simulink model "uGrid_1PH_hd_ATD_prueba"  (R2018a)
settings: Solver=ode45  StartTime=0.0  StopTime=1.5  FixedStep=1e-4  MaxStep=1e-4  RelTol=1e-3
PreLoadFcn:
  | SimulinkInit
InitFcn:
  | SimulinkInit
values from neighbouring files (symbols this model uses):
  Ad = sysd.A    [SimulinkInit.m]
  b = 4.91    [parametros_BIO.m]
  Bd = sysd.B    [SimulinkInit.m]
  C = C1+C2+C3+Cl    (= 0.002654)    [SimulinkInit.m]    (also in parametros_BIO.m = 1)
  C1 = Cd(1,:)    [SimulinkInit.m]
  C2 = Cd(2,:)    [SimulinkInit.m]
  C3 = Cd(3,:)    [SimulinkInit.m]
  C4 = Cd(4,:)    [SimulinkInit.m]
  Cd = sysd.C    [SimulinkInit.m]
  K = 25    [parametros_BIO.m]    (also in uio_linear.m = K1+E*H)
  K1 = 1.15    [SimulinkInit.m]    (also in parametros_BIO.m = 9.66; uio_linear.m = K1')
  K11 = 0.8    [parametros_BIO.m]
  K2 = 1    [SimulinkInit.m]    (also in parametros_BIO.m = 6.97)
  K22 = 0.2    [parametros_BIO.m]
  K3 = 1    [SimulinkInit.m]    (also in parametros_BIO.m = 31.8)
  K33 = 0.23    [parametros_BIO.m]
  K4 = 15.1    [parametros_BIO.m]
  Kd = 0.02    [parametros_BIO.m]
  Kdc = 0.02    [parametros_BIO.m]
  Kf = 1    [parametros_BIO.m]
  Kh = 1.2    [parametros_BIO.m]
  Ks = 21.5    [parametros_BIO.m]
  Ksc = 3    [parametros_BIO.m]
  Kv = 1    [parametros_BIO.m]
  Sbin = 13.8    [parametros_BIO.m]
  Svin = 2.91    [parametros_BIO.m]
  T1 = 0.4    [parametros_BIO.m]
  T2 = 1    [parametros_BIO.m]
  T3 = 15    [parametros_BIO.m]
  T4 = 2.5    [parametros_BIO.m]
  T5 = 3.3    [parametros_BIO.m]
  Tao1 = 0.5    [SimulinkInit.m]
  Tcd = 0.2    [parametros_BIO.m]
  Tcr = 0.01    [parametros_BIO.m]
  Tf = 0.04    [parametros_BIO.m]
  tm = 1e-4    (= 0.0001)    [SimulinkInit.m]
  Tr = 950    [parametros_BIO.m]
  Tt = 450    [parametros_BIO.m]
  Ttd = 0.04    [parametros_BIO.m]
  Tv = 0.05    [parametros_BIO.m]
  V = 20    [parametros_BIO.m]
  wref = 70000    [parametros_BIO.m]
  X_acid = 1.2    [parametros_BIO.m]
  X_meth = 0.35    [parametros_BIO.m]
  Z = 3    [parametros_BIO.m]
undefined symbols (not defined in the file or in its folder): F1, F2, F3, F4, G, GF, H1, H2, H3, H4, Ion, K1U, K2U, K3U, K4U, Lithium, ss1, ss2
libraries: powerlib x58, dsparch4 x12, truetime x12, powerlib_meascontrol x4, simulink x1, electricdrivelib x1
(part 2 of 3)

== system uGrid_1PH_hd_ATD_prueba/CSI_Control_DIESEL ==
  V_measured : Inport
  I_measured : Inport  Port=2
  P_ref : Inport  Port=3
  Q_ref : Inport  Port=4
  Demux : Demux  Outputs=3
  Hw1 : dsparch4/Analog Filter Design  method=Bessel  filttype=Lowpass  N=4  Wlo=30*2*pi  Whi=80  Rp=2  Rs=80
  Hw3 : dsparch4/Analog Filter Design  method=Bessel  filttype=Lowpass  N=4  Wlo=30*2*pi  Whi=80  Rp=2  Rs=80
  Mux : Mux
  TTKernel_DIESEL : truetime/TrueTime Kernel  sfun=DIESEL_init  args=[]  ninputsoutputs=[4 3]  ntriggers=0  trigtype=falling  nwnodenbr=[]  clockoffsetdrift=[0 0]  schedoutput=on  battery=off  poweroutput=off
  D : Outport
  P_measure : Outport  Port=2
  Q_measure : Outport  Port=3
  wires:
  Mux/1 -> TTKernel_DIESEL/1
  Demux/3 -> Hw3/1
  Demux/2 -> Hw1/1
  TTKernel_DIESEL/1 -> Demux/1
  Demux/1 -> D/1
  Hw1/1 -> P_measure/1
  Hw3/1 -> Q_measure/1
  P_ref/1 -> Mux/3
  Q_ref/1 -> Mux/4
  I_measured/1 -> Mux/2
  V_measured/1 -> Mux/1

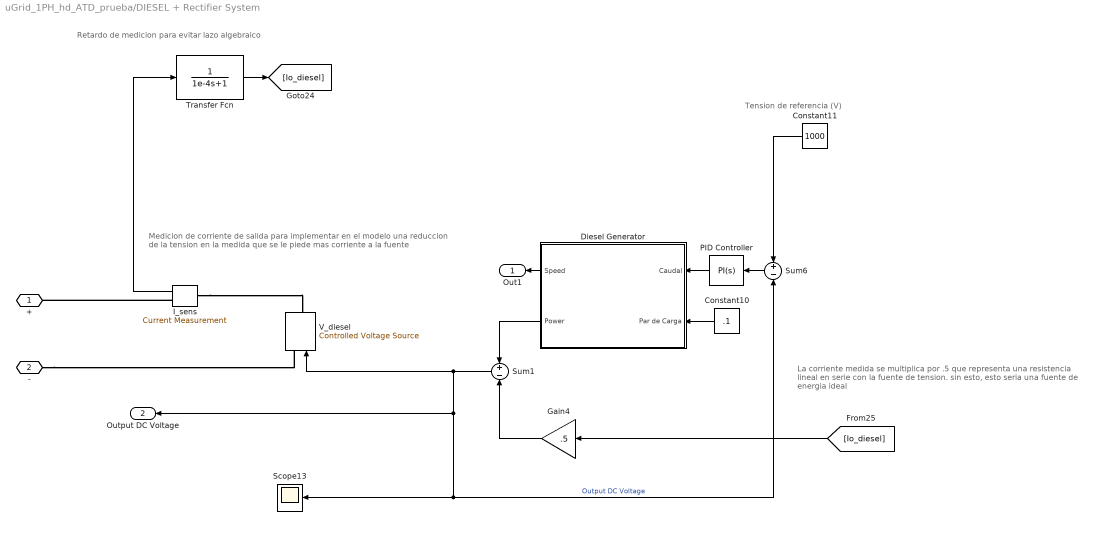
== system uGrid_1PH_hd_ATD_prueba/DIESEL + Rectifier System ==
  note: Tension de referencia (V)
  note: La corriente medida se multiplica por .5 que
      | representa una resistencia lineal en serie con
      | la fuente de tension. sin esto, esto seria una
      | fuente de energia ideal
  note: Medicion de corriente de salida para implementar
      | en el modelo una reduccion de la tension en la
      | medida que se le piede mas corriente a la fuente
  note: Retardo de medicion para evitar lazo algebraico
  Constant10 : Constant  Value=.1
  Constant11 : Constant  Value=1000
  Diesel Generator : Subsystem
  Gain4 : Gain  Gain=.5
  I_sens : powerlib/Measurements/Current Measurement  PhasorSimulation=off  OutputType=Complex  PSBequivalent=0
  PID Controller : simulink/Continuous/PID Controller  Controller=PI  TimeDomain=Continuous-time  SampleTime=-1  IntegratorMethod=Forward Euler  FilterMethod=Forward Euler  Form=Parallel  UseFilter=on  ControllerParametersSource=internal  P=0.00325909628031494  I=0.000326732379168699  D=0.00124823483730586  N=0.606508283225141  InitialConditionSource=internal  InitialConditionForIntegrator=0.248  InitialConditionForFilter=0.24  ExternalReset=none  LimitOutput=off  UpperSaturationLimit=inf  LowerSaturationLimit=-inf  LinearizeAsGain=on  AntiWindupMode=none  Kb=1  TrackingMode=off  Kt=1  PParamMin=[]  PParamMax=[]  IParamMin=[]  IParamMax=[]  DParamMin=[]  DParamMax=[]  NParamMin=[]  NParamMax=[]  KbParamMin=[]  KbParamMax=[]  KtParamMin=[]  KtParamMax=[]  POutMin=[]  POutMax=[]  IOutMin=[]  IOutMax=[]  DOutMin=[]  DOutMax=[]  NOutMin=[]  NOutMax=[]  KbOutMin=[]  KbOutMax=[]  KtOutMin=[]  KtOutMax=[]  IntegratorOutMin=[]  IntegratorOutMax=[]  FilterOutMin=[]  FilterOutMax=[]  SumOutMin=[]  SumOutMax=[]  SumI1OutMin=[]  SumI1OutMax=[]  SumI2OutMin=[]  SumI2OutMax=[]  SumI3OutMin=[]  SumI3OutMax=[]  SumDOutMin=[]  SumDOutMax=[]  SaturationOutMin=[]  SaturationOutMax=[]  IntegratorContinuousStateAttributes=''  IntegratorStateMustResolveToSignalObject=off  IntegratorRTWStateStorageClass=Auto  FilterContinuousStateAttributes=''  FilterStateMustResolveToSignalObject=off  FilterRTWStateStorageClass=Auto  DifferentiatorICPrevScaledInput=0  DifferentiatorOutMin=[]  DifferentiatorOutMax=[]  InitialConditionSetting=State (most efficient)  FilterDiffOutCoefMin=[]  FilterDiffOutCoefMax=[]  SumDenOutMin=[]  SumDenOutMax=[]  SumNumOutMin=[]  SumNumOutMax=[]  ReciprocalOutMin=[]  ReciprocalOutMax=[]  DivideOutMin=[]  DivideOutMax=[]  TunerSelectOption=Transfer Function Based (PID Tuner App)
  Scope13 : Scope
  Sum1 : Sum  Inputs=+-
  Sum6 : Sum  Inputs=+-
  Transfer Fcn : TransferFcn  Denominator=[1e-4 1]
  V_diesel : powerlib/Electrical Sources/Controlled Voltage Source  Initialize=on  Source_Type=AC  Amplitude=0  Phase=0  Frequency=0  Measurements=None
  + : PMIOPort  Side=Left
  - : PMIOPort  Port=2  Side=Left
  Out1 : Outport
  Output DC Voltage : Outport  Port=2
  wires:
  Sum1/1 -> Output DC Voltage/1, Sum6/2, Scope13/1, V_diesel/1  "Output DC Voltage"
  Transfer Fcn/1 -> [Io_diesel]
  I_sens/1 -> Transfer Fcn/1
  Diesel Generator/2(Power) -> Sum1/1
  Sum6/1 -> PID Controller/1
  Diesel Generator/1(Speed) -> Out1/1
  Gain4/1 -> Sum1/2
  Constant10/1 -> Diesel Generator/2(Par de Carga)
  Constant11/1 -> Sum6/1
  [Io_diesel] -> Gain4/1
  PID Controller/1 -> Diesel Generator/1(Caudal)
  connections:
  -/RConn1 -- V_diesel/LConn1
  I_sens/LConn1 -- V_diesel/RConn1
  I_sens/RConn1 -- +/RConn1

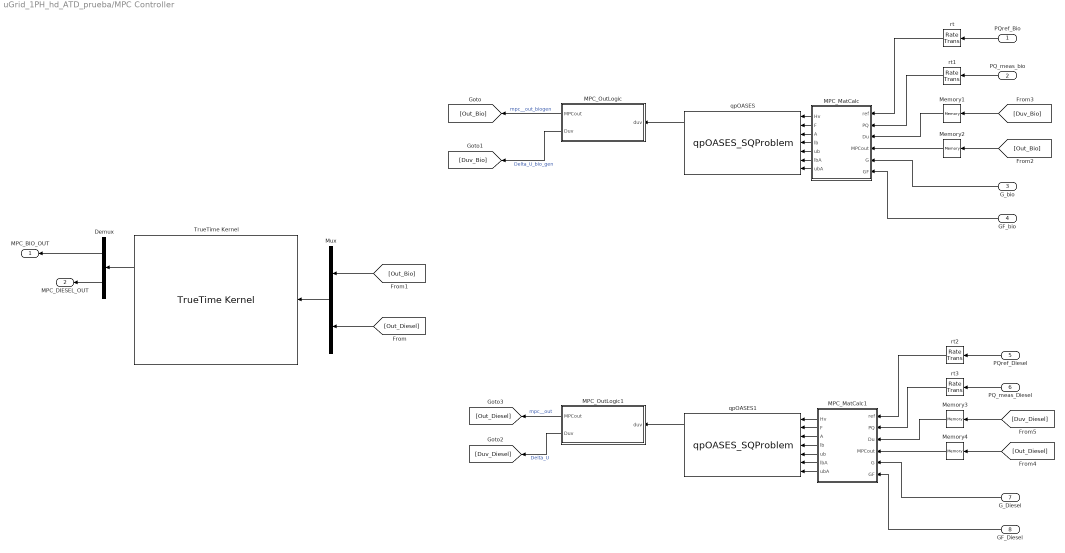
== system uGrid_1PH_hd_ATD_prueba/MPC Controller ==
  PQref_Bio : Inport
  PQ_meas_bio : Inport  Port=2
  G_bio : Inport  Port=3
  GF_bio : Inport  Port=4
  PQref_Diesel : Inport  Port=5
  PQ_meas_Diesel : Inport  Port=6
  G_Diesel : Inport  Port=7
  GF_Diesel : Inport  Port=8
  Demux : Demux  Outputs=2
  MPC_MatCalc : MATLAB Function  TreatAsAtomicUnit=on  SystemSampleTime=1e-3
      settings: MinAlgLoopOccurrences=on
  MPC_MatCalc1 : MATLAB Function  TreatAsAtomicUnit=on  SystemSampleTime=1e-3
      settings: MinAlgLoopOccurrences=on
  MPC_OutLogic : MATLAB Function  TreatAsAtomicUnit=on
      settings: MinAlgLoopOccurrences=on
  MPC_OutLogic1 : MATLAB Function  TreatAsAtomicUnit=on
      settings: MinAlgLoopOccurrences=on
  Memory{1..4} (4 alike) : Memory
  Mux : Mux  Inputs=2
  TrueTime Kernel : truetime/TrueTime Kernel  sfun=MPC_PQ_init  args=[]  ninputsoutputs=[4 4]  ntriggers=0  trigtype=falling  nwnodenbr=[]  clockoffsetdrift=[0 0]  schedoutput=on  battery=off  poweroutput=off
  qpOASES : S-Function  FunctionName=qpOASES_SQProblem  SFunctionDeploymentMode=off  EnableBusSupport=off
  qpOASES1 : S-Function  FunctionName=qpOASES_SQProblem  SFunctionDeploymentMode=off  EnableBusSupport=off
  rt{,1..3} (4 alike) : RateTransition  InitialCondition=[0 0]  OutPortSampleTime=1e-3
  MPC_BIO_OUT : Outport
  MPC_DIESEL_OUT : Outport  Port=2
  wires:
  MPC_MatCalc/7(ubA) -> qpOASES/7
  G_bio/1 -> MPC_MatCalc/5(G)
  MPC_MatCalc/4(lb) -> qpOASES/4
  MPC_MatCalc/6(lbA) -> qpOASES/6
  Memory1/1 -> MPC_MatCalc/3(Du)
  rt1/1 -> MPC_MatCalc/2(PQ)
  GF_bio/1 -> MPC_MatCalc/6(GF)
  PQ_meas_bio/1 -> rt1/1
  MPC_MatCalc/2(F) -> qpOASES/2
  Memory2/1 -> MPC_MatCalc/4(MPCout)
  MPC_MatCalc/5(ub) -> qpOASES/5
  MPC_MatCalc/3(A) -> qpOASES/3
  rt/1 -> MPC_MatCalc/1(ref)
  MPC_MatCalc/1(Hv) -> qpOASES/1
  PQref_Bio/1 -> rt/1
  MPC_MatCalc1/7(ubA) -> qpOASES1/7
  G_Diesel/1 -> MPC_MatCalc1/5(G)
  MPC_MatCalc1/4(lb) -> qpOASES1/4
  MPC_MatCalc1/6(lbA) -> qpOASES1/6
  Memory3/1 -> MPC_MatCalc1/3(Du)
  rt3/1 -> MPC_MatCalc1/2(PQ)
  GF_Diesel/1 -> MPC_MatCalc1/6(GF)
  PQ_meas_Diesel/1 -> rt3/1
  MPC_MatCalc1/2(F) -> qpOASES1/2
  Memory4/1 -> MPC_MatCalc1/4(MPCout)
  MPC_MatCalc1/5(ub) -> qpOASES1/5
  MPC_MatCalc1/3(A) -> qpOASES1/3
  rt2/1 -> MPC_MatCalc1/1(ref)
  MPC_MatCalc1/1(Hv) -> qpOASES1/1
  PQref_Diesel/1 -> rt2/1
  [Duv_Bio] -> Memory1/1
  [Out_Bio] -> Memory2/1
  [Duv_Diesel] -> Memory3/1
  [Out_Diesel] -> Memory4/1
  qpOASES1/1 -> MPC_OutLogic1/1(duv)
  qpOASES/1 -> MPC_OutLogic/1(duv)
  MPC_OutLogic1/2(Duv) -> [Duv_Diesel]  "Delta_U"
  MPC_OutLogic/1(MPCout) -> [Out_Bio]  "mpc__out_biogen"
  MPC_OutLogic1/1(MPCout) -> [Out_Diesel]  "mpc__out"
  Mux/1 -> TrueTime Kernel/1
  MPC_OutLogic/2(Duv) -> [Duv_Bio]  "Delta_U_bio_gen"
  TrueTime Kernel/1 -> Demux/1
  Demux/2 -> MPC_DIESEL_OUT/1
  Demux/1 -> MPC_BIO_OUT/1
  [Out_Diesel] -> Mux/2
  [Out_Bio] -> Mux/1

== system uGrid_1PH_hd_ATD_prueba/MeasureNode_I1 ==
  in : Inport
  Clock : Clock
  MATLAB Function : MATLAB Function  TreatAsAtomicUnit=on
  Pulse Generator1 : DiscretePulseGenerator  PulseType=Time based  Period=1e-4  PulseWidth=50  PhaseDelay=2e-4
  TrueTime Receive : truetime/TrueTime Receive  nwnbr=1  receiver=4  outdim=1  triggeroutput=on  senderoutput=off  lengthoutput=off  priorityoutput=off  timestampoutput=off  signalpoweroutput=off  msgIDoutput=off
  TrueTime Send : truetime/TrueTime Send  trigger=falling  nwnbr=1  sender=3  indim=1  recsource=internal  receiver=4  lengthsource=internal  length=10000  priosource=internal  prio=1  msgIDsource=internal  msgID=0  dynamicSegment=dynamic
  Out : Outport
  wires:
  Pulse Generator1/1 -> TrueTime Send/2
  TrueTime Receive/1 -> Out/1
  Clock/1 -> MATLAB Function/1(u1)
  MATLAB Function/1(y) -> TrueTime Send/1
  in/1 -> MATLAB Function/2(u2)

== system uGrid_1PH_hd_ATD_prueba/MeasureNode_I2 ==
  in : Inport
  Clock : Clock
  Delay : Delay  DelayLength=10
  MATLAB Function : MATLAB Function  TreatAsAtomicUnit=on
  Pulse Generator1 : DiscretePulseGenerator  PulseType=Time based  Period=1e-4  PulseWidth=50  PhaseDelay=1e-4
  TrueTime Receive : truetime/TrueTime Receive  nwnbr=1  receiver=2  outdim=1  triggeroutput=on  senderoutput=off  lengthoutput=off  priorityoutput=off  timestampoutput=off  signalpoweroutput=off  msgIDoutput=off
  TrueTime Send : truetime/TrueTime Send  trigger=falling  nwnbr=1  sender=1  indim=1  recsource=internal  receiver=2  lengthsource=internal  length=10000  priosource=internal  prio=1  msgIDsource=internal  msgID=0  dynamicSegment=dynamic
  Out : Outport
  wires:
  TrueTime Receive/1 -> Out/1
  Pulse Generator1/1 -> TrueTime Send/2
  Clock/1 -> MATLAB Function/1(u1)
  MATLAB Function/1(y) -> TrueTime Send/1
  in/1 -> Delay/1, MATLAB Function/2(u2)
  Delay/1 -> MATLAB Function/3(u3)

== system uGrid_1PH_hd_ATD_prueba/MeasureNode_I3 ==
  in : Inport
  Clock : Clock
  MATLAB Function : MATLAB Function  TreatAsAtomicUnit=on
  Pulse Generator1 : DiscretePulseGenerator  PulseType=Time based  Period=1e-4  PulseWidth=50  PhaseDelay=3e-4
  TrueTime Receive : truetime/TrueTime Receive  nwnbr=1  receiver=6  outdim=1  triggeroutput=on  senderoutput=off  lengthoutput=off  priorityoutput=off  timestampoutput=off  signalpoweroutput=off  msgIDoutput=off
  TrueTime Send : truetime/TrueTime Send  trigger=falling  nwnbr=1  sender=5  indim=1  recsource=internal  receiver=6  lengthsource=internal  length=10000  priosource=internal  prio=1  msgIDsource=internal  msgID=0  dynamicSegment=dynamic
  Out : Outport
  wires:
  in/1 -> MATLAB Function/2(u2)
  Pulse Generator1/1 -> TrueTime Send/2
  TrueTime Receive/1 -> Out/1
  Clock/1 -> MATLAB Function/1(u1)
  MATLAB Function/1(y) -> TrueTime Send/1

== system uGrid_1PH_hd_ATD_prueba/MeasureNode_I4 ==
  in : Inport
  Clock : Clock
  MATLAB Function : MATLAB Function  TreatAsAtomicUnit=on
  Pulse Generator1 : DiscretePulseGenerator  PulseType=Time based  Period=1e-4  PulseWidth=50  PhaseDelay=4e-4
  TrueTime Receive : truetime/TrueTime Receive  nwnbr=1  receiver=8  outdim=1  triggeroutput=on  senderoutput=off  lengthoutput=off  priorityoutput=off  timestampoutput=off  signalpoweroutput=off  msgIDoutput=off
  TrueTime Send : truetime/TrueTime Send  trigger=falling  nwnbr=1  sender=7  indim=1  recsource=internal  receiver=8  lengthsource=internal  length=10000  priosource=internal  prio=1  msgIDsource=internal  msgID=0  dynamicSegment=dynamic
  Out : Outport
  wires:
  Pulse Generator1/1 -> TrueTime Send/2
  TrueTime Receive/1 -> Out/1
  in/1 -> MATLAB Function/2(u2)
  MATLAB Function/1(y) -> TrueTime Send/1
  Clock/1 -> MATLAB Function/1(u1)

== system uGrid_1PH_hd_ATD_prueba/Subsystem ==
  Battery : electricdrivelib/Extra Sources/Battery  BatType=Lithium-Ion  ShowTempParam=off  ThermalPreset=no  ShowAgeParam=off  NomV=1000  NomQ=20  SOC=100  Batt_Tr=10e-3  PresetModel=off  MaxQ=1  MinV=825  FullV=1280.3859  Dis_rate=200  R=50e-3  Normal_OP=0.90435  expZone="[1188.4244    0.049130435]"  current=[6.5 13 32.5 50]  Units=Time  Tci=20  NomT=20  T2=-30  MaxQ2=4.8  FullV2=7.1  Normal_OP2=5.655  expZone2="[6.58           1]"  Rca=0.6  ti=2000  Dp=0  Neq0=0  Tsim=1e6  Ta1=25  Qeol=5.4*0.9  Reol=0.013333*1.2  Char_age=[2.3478, 3]  Dis_age=[2.3478, 10]  N1=1500  N2=10500  N3=1000  N4=1400  Ta2=45  N5=950
  Constant2 : Constant  Value=1000
  Constant4 : Constant  Value=25
  Controlled Current Source : powerlib/Electrical Sources/Controlled Current Source  Initialize=on  Source_Type=AC  Amplitude=0  Phase=0  Frequency=0  Measurements=None
  Gain3 : Gain  Gain=1/10
  PV panel1 : Subsystem
      mask Display: image('panel.jpg')
  Rcable : powerlib/Elements/Series RLC Branch  LConnTagsString=__new0  RConnTagsString=__new0  BranchType=R  Resistance=1e-3  Inductance=1e-3  SetiL0=off  InitialCurrent=0  Capacitance=1e-6  Setx0=off  InitialVoltage=0  Measurements=None
  Rin2 : powerlib/Elements/Series RLC Branch  LConnTagsString=__new0  RConnTagsString=__new0  BranchType=C  Resistance=.001  Inductance=0  SetiL0=off  InitialCurrent=0  Capacitance=1000e-6  Setx0=off  InitialVoltage=0  Measurements=None
  + : PMIOPort  Side=Left
  - : PMIOPort  Port=2  Side=Left
  Out1 : Outport
  wires:
  PV panel1/1(I) -> Gain3/1
  Gain3/1 -> Controlled Current Source/1
  Battery/1 -> Out1/1
  Constant4/1 -> PV panel1/3(Top)
  Constant2/1 -> PV panel1/2(G)
  [V] -> PV panel1/1(V)
  connections:
  Rcable/RConn1 -- +/RConn1
  Battery/LConn1 -- Controlled Current Source/RConn1 -- Rcable/LConn1 -- Rin2/LConn1
  Battery/LConn2 -- -/RConn1 -- Rin2/RConn1 -- Controlled Current Source/LConn1

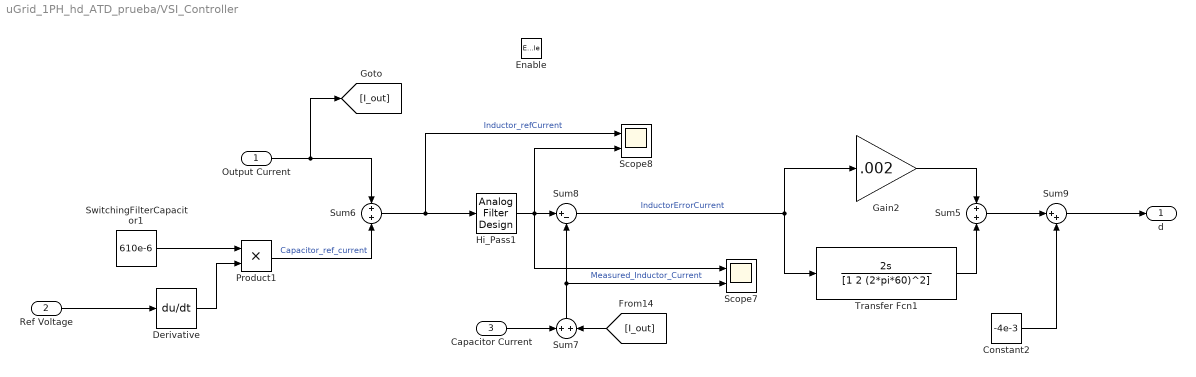
== system uGrid_1PH_hd_ATD_prueba/VSI_Controller ==
  Output Current : Inport
  Ref Voltage : Inport  Port=2
  Capacitor Current : Inport  Port=3
  Enable : EnablePort
  Constant2 : Constant  Value=-4e-3
  Derivative : Derivative  CoefficientInTFapproximation=1e-3
  Gain2 : Gain  Gain=.002
  Hi_Pass1 : dsparch4/Analog Filter Design  method=Bessel  filttype=Highpass  N=1  Wlo=1*2*pi  Whi=80  Rp=2  Rs=40
  Product1 : Product
  Scope7 : Scope  NumInputPorts=2
  Scope8 : Scope  NumInputPorts=2
  Sum5 : Sum  Inputs=+|+
  Sum6 : Sum  Inputs=+|+
  Sum7 : Sum  Inputs=+|+
  Sum8 : Sum  Inputs=|+-
  Sum9 : Sum  Inputs=|++
  SwitchingFilterCapacitor1 : Constant  Value=610e-6
  Transfer Fcn1 : TransferFcn  Numerator=[2 0]  Denominator=[1 2 (2*pi*60)^2]
  d : Outport
  wires:
  Derivative/1 -> Product1/2
  Sum6/1 -> Hi_Pass1/1, Scope8/1  "Inductor_refCurrent"
  Sum8/1 -> Transfer Fcn1/1, Gain2/1  "InductorErrorCurrent"
  Ref Voltage/1 -> Derivative/1
  Constant2/1 -> Sum9/2
  Capacitor Current/1 -> Sum7/1
  Transfer Fcn1/1 -> Sum5/2
  Output Current/1 -> Sum6/1, [I_out]
  [I_out] -> Sum7/2
  Gain2/1 -> Sum5/1
  SwitchingFilterCapacitor1/1 -> Product1/1
  Hi_Pass1/1 -> Scope8/2, Sum8/1, Scope7/1
  Product1/1 -> Sum6/2  "Capacitor_ref_current"
  Sum9/1 -> d/1
  Sum5/1 -> Sum9/1
  Sum7/1 -> Scope7/2, Sum8/2  "Measured_Inductor_Current"

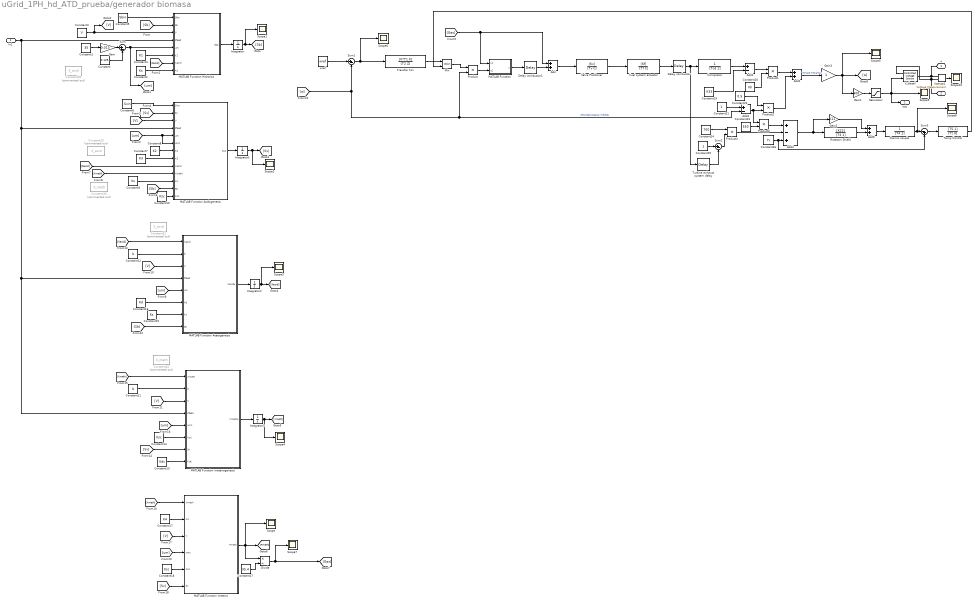
== system uGrid_1PH_hd_ATD_prueba/generador biomasa ==
  In1 : Inport
  Add : Sum
  Add1 : Sum  Inputs=+-
  Add2 : Sum
  Add3 : Sum  Inputs=+-
  Add4 : Sum  Inputs=+-+
  Add5 : Sum
  Compresor : TransferFcn  Denominator=[Tcd 1]
  Constant : Constant  Value=0.129
  Constant1 : Constant  Value=35
  Constant10 : Constant  Value=Ksc
  Constant11 : Constant  Value=b
  Constant12 : Constant  Value=b
  Constant13 : Constant  Value=Kdc
  Constant14 : Constant  Value=Ksc
  Constant15 : Constant  Value=Ks
  Constant16 : Constant  Value=Kd
  Constant17 : Constant  Value=K4
  Constant18 : Constant  Value=Ksc
  Constant19 : Constant  Value=K33
  Constant2 : Constant  Value=Ks
  Constant20 : Constant  Value=Kh
  Constant21 : Constant
  Constant22 : Constant  Value=0.5
  Constant23 : Constant  Value=550
  Constant24 : Constant  Value=700
  Constant25 : Constant
  Constant26 : Constant  Value=Tr
  Constant27 : Constant  Value=35.4
  Constant28 : Constant  Commented=on  Value=X_acid
  Constant29 : Constant  Commented=on  Value=X_acid
  Constant3 : Constant  Value=V
  Constant30 : Constant  Commented=on  Value=X_meth
  Constant31 : Constant  Commented=on  Value=X_acid
  Constant32 : Constant  Commented=on  Value=X_meth
  Constant4 : Constant  Value=K1
  Constant5 : Constant  Value=Sbin
  Constant6 : Constant  Value=Svin
  Constant7 : Constant  Value=K3
  Constant8 : Constant  Value=K2
  Constant9 : Constant  Value=Ks
  Delay combustor : TransportDelay  DelayTime=Tcr
  Delay combustor1 : TransportDelay  DelayTime=0
  Divide : Product  Inputs=*/
  Fuel system actuator : TransferFcn  Numerator=[Kf]  Denominator=[Tf C]
  Gain : Gain  Gain=0.013
  Gain1 : Gain  Gain=900
  Gain2 : Gain  Gain=K11
  Gain3 : Gain
  Integrator : Integrator
  Integrator1 : Integrator
  Integrator2 : Integrator  InitialCondition=1.2
  Integrator3 : Integrator  InitialCondition=0.35
  MATLAB Function : MATLAB Function  TreatAsAtomicUnit=on
  MATLAB Function Acetogenesis : MATLAB Function  TreatAsAtomicUnit=on
  MATLAB Function Acidogenesis : MATLAB Function  TreatAsAtomicUnit=on
  MATLAB Function Hidrolisis : MATLAB Function  TreatAsAtomicUnit=on
  MATLAB Function metano : MATLAB Function  TreatAsAtomicUnit=on
  MATLAB Function metanogenesis : MATLAB Function  TreatAsAtomicUnit=on
  Min : MinMax  Inputs=2
  Product{,1..4} (5 alike) : Product
  Rotation Shield : TransferFcn  Numerator=[K22]  Denominator=[T3 1]
  Saturation : Saturate  UpperLimit=1000  LowerLimit=0
  Scope{,1..10} (11 alike) : Scope
  Sum : Sum  Inputs=|+-
  Sum1 : Sum  Inputs=|+-
  Sum2 : Sum  Inputs=|+-
  Sum3 : Sum  Inputs=|-+
  Temp Control : TransferFcn  Numerator=[T5 1]  Denominator=[Tt 0]
  Transfer Fcn : TransferFcn  Numerator=[K*T1 K]  Denominator=[T2 Z]
  Turbine exhaust system delay : TransportDelay  DelayTime=Ttd
  V_diesel : powerlib/Electrical Sources/Controlled Voltage Source  Initialize=on  Source_Type=DC  Amplitude=0  Phase=0  Frequency=0  Measurements=None
  Valve Positioner : TransferFcn  Numerator=[Kv]  Denominator=[Tv C]
  Vsensa1 : powerlib/Measurements/Voltage Measurement  PhasorSimulation=off  OutputType=Complex  PSBequivalent=0
  thermo couple : TransferFcn  Denominator=[T4 1]
  wref : Constant  Value=wref
  + : PMIOPort  Side=Left
  - : PMIOPort  Port=2  Side=Left
  Vdc : Outport
  wires:
  MATLAB Function metano/1(Fmeth) -> Divide/1, Scope/1, [Fmeth]
  Sum/1 -> [um], MATLAB Function Hidrolisis/5(um)
  Constant16/1 -> MATLAB Function Acetogenesis/6(Kd)
  Temp Control/1 -> Min/2
  Integrator/1 -> Scope1/1, [Sb]
  Gain3/1 -> Gain1/1, Scope5/1, [w]
  Sum1/1 -> Transfer Fcn/1, Scope6/1
  [Sb] -> MATLAB Function Acetogenesis/8(Sb)
  [Sv] -> MATLAB Function metanogenesis/7(Sv)
  Add4/1 -> Rotation Shield/1, Gain2/1
  Constant8/1 -> MATLAB Function Acidogenesis/7(K2)
  Constant24/1 -> Product4/1
  [V] -> MATLAB Function Acetogenesis/3(V)
  Constant23/1 -> Product3/2
  Constant27/1 -> Divide/2
  [Sb] -> MATLAB Function Acidogenesis/12(Sb)
  Integrator3/1 -> Scope4/1, [Xmeth]
  Integrator2/1 -> Scope3/1, [Xacid]
  Divide/1 -> Scope7/1, [Gas]
  Constant7/1 -> MATLAB Function Acidogenesis/8(K3)
  Delay combustor/1 -> Turbine exhaust system delay/1, Compresor/1
  [V] -> MATLAB Function Acidogenesis/3(V)
  Constant12/1 -> MATLAB Function Acetogenesis/2(b)
  Sum2/1 -> Product4/2
  [V] -> MATLAB Function metanogenesis/3(V)
  Gain/1 -> Sum/1
  Product/1 -> MATLAB Function/2(u2)
  [w] -> Product/2, Add3/2, Sum1/2  "velocidad angular medida"
  Constant6/1 -> MATLAB Function Acidogenesis/1(Svin)
  wref/1 -> Sum1/1
  [Gas] -> MATLAB Function/1(u1), Add/1
  [Sv] -> MATLAB Function metano/6(Sv)
  MATLAB Function Hidrolisis/1(Sbp) -> Integrator/1
  Turbine exhaust system delay/1 -> Sum2/2
  MATLAB Function Acetogenesis/1(Xacidp) -> Integrator2/1
  Constant/1 -> Sum/2
  Constant18/1 -> MATLAB Function metano/5(Ksc)
  In1/1 -> MATLAB Function Acidogenesis/4(Ffeed), MATLAB Function metanogenesis/4(Ffeed), MATLAB Function Acetogenesis/4(Ffeed), MATLAB Function Hidrolisis/4(Ffeed)
  Add3/1 -> Product3/1, Product2/2
  [um] -> MATLAB Function Acetogenesis/5(um)
  Product3/1 -> Add4/1
  Constant15/1 -> MATLAB Function Acetogenesis/7(Ks)
  thermo couple/1 -> Scope8/1, Sum3/1
  Fuel system actuator/1 -> Delay combustor/1
  Add/1 -> Valve Positioner/1
  Add5/1 -> thermo couple/1
  Gain2/1 -> Add5/1
  Constant22/1 -> Product2/1
  [um] -> MATLAB Function metano/4(umc)
  Compresor/1 -> Add1/1
  Constant10/1 -> MATLAB Function Acidogenesis/13(Ksc)
  [um] -> MATLAB Function Acidogenesis/6(umc), MATLAB Function Acidogenesis/5(um)
  Constant9/1 -> MATLAB Function Acidogenesis/11(Ks)
  Constant1/1 -> Gain/1
  Constant13/1 -> MATLAB Function metanogenesis/8(Kdc)
  Constant26/1 -> Sum3/2, Add4/3
  Integrator1/1 -> Scope2/1, [Sv]
  [Xmeth] -> MATLAB Function metanogenesis/1(Xmeth)
  Add2/1 -> Gain3/1  "Torque mecánico"
  MATLAB Function/1(y) -> Delay combustor1/1
  Saturation/1 -> Vdc/1, V_diesel/1, Scope9/1
  [Sb] -> MATLAB Function Hidrolisis/2(Sb)
  Min/1 -> Product/1
  Constant3/1 -> [V], MATLAB Function Hidrolisis/3(V)
  MATLAB Function Acidogenesis/1(Svp) -> Integrator1/1
  Constant5/1 -> MATLAB Function Hidrolisis/1(Sbin)
  Constant20/1 -> Product1/2
  [Xmeth] -> MATLAB Function Acidogenesis/10(Xmeth)
  Sum3/1 -> Temp Control/1
  Gain1/1 -> Saturation/1
  Constant21/1 -> Add3/1
  Constant25/1 -> Sum2/1
  Product2/1 -> Add2/2
  [Xacid] -> MATLAB Function Acidogenesis/9(Xacid)
  Valve Positioner/1 -> Fuel system actuator/1
  Constant4/1 -> MATLAB Function Hidrolisis/6(K1)
  Constant11/1 -> MATLAB Function metanogenesis/2(b)
  Rotation Shield/1 -> Add5/2
  Add1/1 -> Product1/1
  [Sv] -> MATLAB Function Acidogenesis/2(Sv)
  [Xacid] -> MATLAB Function Acetogenesis/1(Xacid)
  Constant19/1 -> Add1/2
  Product1/1 -> Add2/1
  Transfer Fcn/1 -> Min/1
  Delay combustor1/1 -> Add/2
  [um] -> MATLAB Function metanogenesis/5(umc)
  MATLAB Function metanogenesis/1(Xmethp) -> Integrator3/1
  Constant14/1 -> MATLAB Function metanogenesis/6(Ksc)
  Product4/1 -> Add4/2
  Constant2/1 -> MATLAB Function Hidrolisis/8(Ks)
  Constant17/1 -> MATLAB Function metano/2(K4)
  [V] -> MATLAB Function metano/3(V)
  [Xmeth] -> MATLAB Function metano/1(Xmeth)
  [Xacid] -> MATLAB Function Hidrolisis/7(Xacid)
  Vsensa1/1 -> Scope10/1
  connections:
  V_diesel/RConn1 -- Vsensa1/LConn1 -- +/RConn1
  V_diesel/LConn1 -- Vsensa1/LConn2 -- -/RConn1

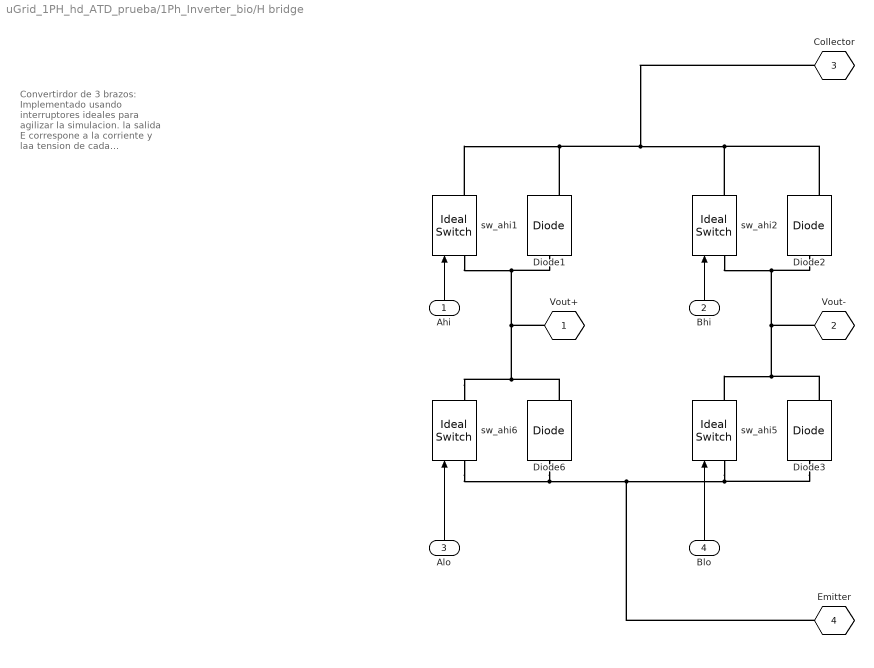
== system uGrid_1PH_hd_ATD_prueba/1Ph_Inverter_bio/H bridge ==
  note: Convertirdor de 3 brazos:
      |
      | Implementado usando interruptores
      | ideales para agilizar la simulacion.
      | la salida E correspone a la corriente y laa
      | tension de cada componente
      | (sea interruptor o diodo) y su respectiva
      | corriente. no tienen puerto de salida ya que no
      | son relevantes para lo que se desea simular.
      |
      | si g=0 interruptor no conduce.
      | si g=1 interruptor conduce.
      |
      | conmutacion ocurre instantaneamente sin
      | retardo.
  Ahi : Inport
  Bhi : Inport  Port=2
  Alo : Inport  Port=3
  Blo : Inport  Port=4
   sw_ahi{1..2,5..6} (4 alike) : powerlib/Power Electronics/Ideal Switch  Ron=0.1  Lon=0  IC=0  Rs=1e6  Cs=10e-12  Measurements=on
  Diode{1..3,6} (4 alike) : powerlib/Power Electronics/Diode  Ron=.2  Lon=0  Vf=0.8  IC=0  UseSnubber=0  Rs=0  Cs=0  Measurements=on
  " Vout+" : PMIOPort  Tag=PMCPort  Side=Right
  Vout- : PMIOPort  Tag=PMCPort  Port=2  Side=Right
  Collector : PMIOPort  Tag=PMCPort  Port=3  Side=Right
  Emitter : PMIOPort  Tag=PMCPort  Port=4  Side=Right
  wires:
  Alo/1 -> " sw_ahi6"/1
  Ahi/1 -> " sw_ahi1"/1
  Blo/1 -> " sw_ahi5"/1
  Bhi/1 -> " sw_ahi2"/1
  connections:
  Diode3/RConn1 -- Vout-/RConn1 -- " sw_ahi2"/LConn1 -- Diode2/LConn1 -- " sw_ahi5"/RConn1
  Diode3/LConn1 -- Emitter/RConn1 -- Diode6/LConn1 -- " sw_ahi6"/LConn1 -- " sw_ahi5"/LConn1
  Diode2/RConn1 -- Collector/RConn1 -- " sw_ahi1"/RConn1 -- Diode1/RConn1 -- " sw_ahi2"/RConn1
  " sw_ahi6"/RConn1 -- Diode6/RConn1 -- " Vout+"/RConn1 -- Diode1/LConn1 -- " sw_ahi1"/LConn1

== system uGrid_1PH_hd_ATD_prueba/1Ph_Inverter_bio/Io_measure ==
  A_current : Inport
  Enable : EnablePort
  Hw1 : dsparch4/Analog Filter Design  method=Bessel  filttype=Lowpass  N=2  Wlo=7000*2*pi  Whi=80  Rp=2  Rs=80
  Transfer Fcn : TransferFcn  Denominator=[1e-6 1]
  Out1 : Outport
  wires:
  Transfer Fcn/1 -> Hw1/1
  A_current/1 -> Transfer Fcn/1
  Hw1/1 -> Out1/1

== system uGrid_1PH_hd_ATD_prueba/1Ph_Inverter_bio/Subsystem ==
  Din : Inport
  Enable : EnablePort
  Gain : Gain  Gain=15
  PWM Generator (DC-DC) : powerlib_meascontrol/Pulse & Signal Generators/PWM Generator (DC-DC)  Fsw=f_sw  Ts=samp_f
  Steper1 : Subsystem
  Steper3 : Subsystem
  not_pwm : MATLAB Function  TreatAsAtomicUnit=on
  nPWM : Outport
  PWM : Outport  Port=2
  wires:
  not_pwm/1(y) -> Steper3/1(In1)
  Steper3/1(Out1) -> nPWM/1
  Gain/1 -> Steper1/1(In1), not_pwm/1(u)
  Din/1 -> PWM Generator (DC-DC)/1
  PWM Generator (DC-DC)/1 -> Gain/1
  Steper1/1(Out1) -> PWM/1

== system uGrid_1PH_hd_ATD_prueba/1Ph_Inverter_bio/Subsystem1 ==
  A_volts : Inport
  Enable : EnablePort
  Hw4 : dsparch4/Analog Filter Design  method=Bessel  filttype=Lowpass  N=2  Wlo=7000*2*pi  Whi=80  Rp=2  Rs=80
  Transfer Fcn1 : TransferFcn  Denominator=[1e-6 1]
  Out1 : Outport
  wires:
  A_volts/1 -> Transfer Fcn1/1
  Transfer Fcn1/1 -> Hw4/1
  Hw4/1 -> Out1/1

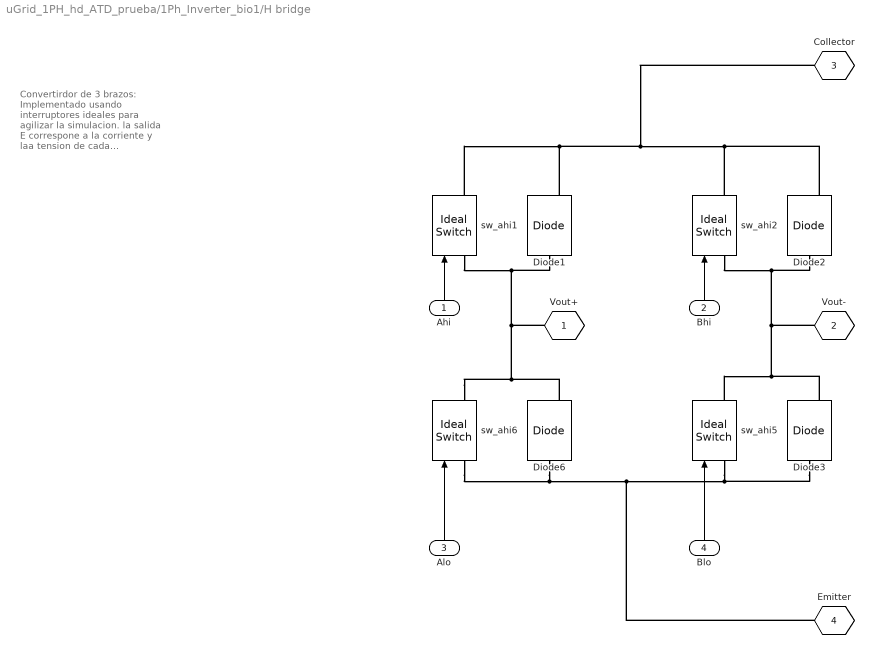
== system uGrid_1PH_hd_ATD_prueba/1Ph_Inverter_bio1/H bridge ==
  note: Convertirdor de 3 brazos:
      |
      | Implementado usando interruptores
      | ideales para agilizar la simulacion.
      | la salida E correspone a la corriente y laa
      | tension de cada componente
      | (sea interruptor o diodo) y su respectiva
      | corriente. no tienen puerto de salida ya que no
      | son relevantes para lo que se desea simular.
      |
      | si g=0 interruptor no conduce.
      | si g=1 interruptor conduce.
      |
      | conmutacion ocurre instantaneamente sin
      | retardo.
  Ahi : Inport
  Bhi : Inport  Port=2
  Alo : Inport  Port=3
  Blo : Inport  Port=4
   sw_ahi{1..2,5..6} (4 alike) : powerlib/Power Electronics/Ideal Switch  Ron=0.1  Lon=0  IC=0  Rs=1e6  Cs=10e-12  Measurements=on
  Diode{1..3,6} (4 alike) : powerlib/Power Electronics/Diode  Ron=.2  Lon=0  Vf=0.8  IC=0  UseSnubber=0  Rs=0  Cs=0  Measurements=on
  " Vout+" : PMIOPort  Tag=PMCPort  Side=Right
  Vout- : PMIOPort  Tag=PMCPort  Port=2  Side=Right
  Collector : PMIOPort  Tag=PMCPort  Port=3  Side=Right
  Emitter : PMIOPort  Tag=PMCPort  Port=4  Side=Right
  wires:
  Alo/1 -> " sw_ahi6"/1
  Ahi/1 -> " sw_ahi1"/1
  Blo/1 -> " sw_ahi5"/1
  Bhi/1 -> " sw_ahi2"/1
  connections:
  Diode3/RConn1 -- Vout-/RConn1 -- " sw_ahi2"/LConn1 -- Diode2/LConn1 -- " sw_ahi5"/RConn1
  Diode3/LConn1 -- Emitter/RConn1 -- Diode6/LConn1 -- " sw_ahi6"/LConn1 -- " sw_ahi5"/LConn1
  Diode2/RConn1 -- Collector/RConn1 -- " sw_ahi1"/RConn1 -- Diode1/RConn1 -- " sw_ahi2"/RConn1
  " sw_ahi6"/RConn1 -- Diode6/RConn1 -- " Vout+"/RConn1 -- Diode1/LConn1 -- " sw_ahi1"/LConn1

== system uGrid_1PH_hd_ATD_prueba/1Ph_Inverter_bio1/Ic Measure ==
  Ic : Inport
  Enable : EnablePort
  Hw5 : dsparch4/Analog Filter Design  method=Bessel  filttype=Lowpass  N=2  Wlo=7000*2*pi  Whi=80  Rp=2  Rs=80
  Transfer Fcn2 : TransferFcn  Denominator=[1e-6 1]
  Out1 : Outport
  wires:
  Transfer Fcn2/1 -> Hw5/1
  Ic/1 -> Transfer Fcn2/1
  Hw5/1 -> Out1/1

== system uGrid_1PH_hd_ATD_prueba/1Ph_Inverter_bio1/Io_measure ==
  A_current : Inport
  Enable : EnablePort
  Hw2 : dsparch4/Analog Filter Design  method=Bessel  filttype=Lowpass  N=2  Wlo=7000*2*pi  Whi=80  Rp=2  Rs=80
  Transfer Fcn : TransferFcn  Denominator=[1e-6 1]
  Out1 : Outport
  wires:
  Transfer Fcn/1 -> Hw2/1
  Hw2/1 -> Out1/1
  A_current/1 -> Transfer Fcn/1

== system uGrid_1PH_hd_ATD_prueba/1Ph_Inverter_bio1/Steper1 ==
  In1 : Inport
  Product : Product
  Step : Step  Time=st_time  SampleTime=samp_f
  Out1 : Outport
  wires:
  Step/1 -> Product/2
  In1/1 -> Product/1
  Product/1 -> Out1/1

== system uGrid_1PH_hd_ATD_prueba/1Ph_Inverter_bio1/Steper3 ==
  In1 : Inport
  Product : Product
  Step : Step  Time=st_time  SampleTime=samp_f
  Out1 : Outport
  wires:
  Product/1 -> Out1/1
  In1/1 -> Product/1
  Step/1 -> Product/2

== system uGrid_1PH_hd_ATD_prueba/1Ph_Inverter_bio1/Vo_measure ==
  A_volts : Inport
  Enable : EnablePort
  Hw6 : dsparch4/Analog Filter Design  method=Bessel  filttype=Lowpass  N=2  Wlo=7000*2*pi  Whi=80  Rp=2  Rs=80
  Transfer Fcn1 : TransferFcn  Denominator=[1e-6 1]
  Out1 : Outport
  wires:
  Transfer Fcn1/1 -> Hw6/1
  Hw6/1 -> Out1/1
  A_volts/1 -> Transfer Fcn1/1

== system uGrid_1PH_hd_ATD_prueba/1Ph_Inverter_diesel/H bridge ==
  note: Convertirdor de 3 brazos:
      |
      | Implementado usando interruptores
      | ideales para agilizar la simulacion.
      | la salida E correspone a la corriente y laa
      | tension de cada componente
      | (sea interruptor o diodo) y su respectiva
      | corriente. no tienen puerto de salida ya que no
      | son relevantes para lo que se desea simular.
      |
      | si g=0 interruptor no conduce.
      | si g=1 interruptor conduce.
      |
      | conmutacion ocurre instantaneamente sin
      | retardo.
  Ahi : Inport
  Bhi : Inport  Port=2
  Alo : Inport  Port=3
  Blo : Inport  Port=4
   sw_ahi{1..2,5..6} (4 alike) : powerlib/Power Electronics/Ideal Switch  Ron=0.1  Lon=0  IC=0  Rs=1e6  Cs=10e-12  Measurements=on
  Diode{1..3,6} (4 alike) : powerlib/Power Electronics/Diode  Ron=.2  Lon=0  Vf=0.8  IC=0  UseSnubber=0  Rs=0  Cs=0  Measurements=on
  " Vout+" : PMIOPort  Tag=PMCPort  Side=Right
  Vout- : PMIOPort  Tag=PMCPort  Port=2  Side=Right
  Collector : PMIOPort  Tag=PMCPort  Port=3  Side=Right
  Emitter : PMIOPort  Tag=PMCPort  Port=4  Side=Right
  wires:
  Bhi/1 -> " sw_ahi2"/1
  Blo/1 -> " sw_ahi5"/1
  Ahi/1 -> " sw_ahi1"/1
  Alo/1 -> " sw_ahi6"/1
  connections:
  " sw_ahi1"/LConn1 -- Diode1/LConn1 -- " Vout+"/RConn1 -- Diode6/RConn1 -- " sw_ahi6"/RConn1
  " sw_ahi2"/RConn1 -- Diode1/RConn1 -- " sw_ahi1"/RConn1 -- Collector/RConn1 -- Diode2/RConn1
  " sw_ahi5"/LConn1 -- " sw_ahi6"/LConn1 -- Diode6/LConn1 -- Emitter/RConn1 -- Diode3/LConn1
  " sw_ahi5"/RConn1 -- Diode2/LConn1 -- " sw_ahi2"/LConn1 -- Vout-/RConn1 -- Diode3/RConn1

== system uGrid_1PH_hd_ATD_prueba/1Ph_Inverter_diesel/Io_measure ==
  A_current : Inport
  Enable : EnablePort
  Hw7 : dsparch4/Analog Filter Design  method=Bessel  filttype=Lowpass  N=2  Wlo=7000*2*pi  Whi=80  Rp=2  Rs=80
  Transfer Fcn : TransferFcn  Denominator=[1e-6 1]
  Out1 : Outport
  wires:
  Hw7/1 -> Out1/1
  Transfer Fcn/1 -> Hw7/1
  A_current/1 -> Transfer Fcn/1

== system uGrid_1PH_hd_ATD_prueba/1Ph_Inverter_diesel/Subsystem ==
  Din : Inport
  Enable : EnablePort
  Gain : Gain  Gain=15
  PWM Generator (DC-DC) : powerlib_meascontrol/Pulse & Signal Generators/PWM Generator (DC-DC)  Fsw=f_sw  Ts=samp_f
  Steper1 : Subsystem
  Steper3 : Subsystem
  not_pwm : MATLAB Function  TreatAsAtomicUnit=on
  nPWM : Outport
  PWM : Outport  Port=2
  wires:
  PWM Generator (DC-DC)/1 -> Gain/1
  Gain/1 -> not_pwm/1(u), Steper1/1(In1)
  Din/1 -> PWM Generator (DC-DC)/1
  not_pwm/1(y) -> Steper3/1(In1)
  Steper3/1(Out1) -> nPWM/1
  Steper1/1(Out1) -> PWM/1

== system uGrid_1PH_hd_ATD_prueba/1Ph_Inverter_diesel/Vo_measure ==
  A_volts : Inport
  Enable : EnablePort
  Hw3 : dsparch4/Analog Filter Design  method=Bessel  filttype=Lowpass  N=2  Wlo=7000*2*pi  Whi=80  Rp=2  Rs=80
  Transfer Fcn1 : TransferFcn  Denominator=[1e-6 1]
  Out1 : Outport
  wires:
  Transfer Fcn1/1 -> Hw3/1
  Hw3/1 -> Out1/1
  A_volts/1 -> Transfer Fcn1/1

== system uGrid_1PH_hd_ATD_prueba/DIESEL + Rectifier System/Diesel Generator ==
  Caudal : Inport
  Par de Carga : Inport  Port=2
  " 1" : Gain  Gain=1.15
  " Generador1" : Gain  Gain=1/2
  Gain1 : Gain  Gain=12000
  Motor de Combustión1 : TransportDelay  DelayTime=Tao1
  State-Space : StateSpace  A=ss1.A  B=ss1.B  C=ss1.C  D=ss1.D  InitialCondition=0.17566/ss1.C
  State-Space1 : StateSpace  A=ss2.A  B=ss2.B  C=ss2.C  D=ss2.D  InitialCondition=0.2493/ss2.C
  Sum2 : Sum  Inputs=|+-
  Speed : Outport
  Power : Outport  Port=2
  wires:
  " 1"/1 -> Motor de Combustión1/1
  " Generador1"/1 -> Gain1/1
  Motor de Combustión1/1 -> Sum2/1
  State-Space1/1 -> " 1"/1
  State-Space/1 -> Speed/1, " Generador1"/1  "Velocidad"
  Sum2/1 -> State-Space/1
  Caudal/1 -> State-Space1/1
  Par de Carga/1 -> Sum2/2
  Gain1/1 -> Power/1

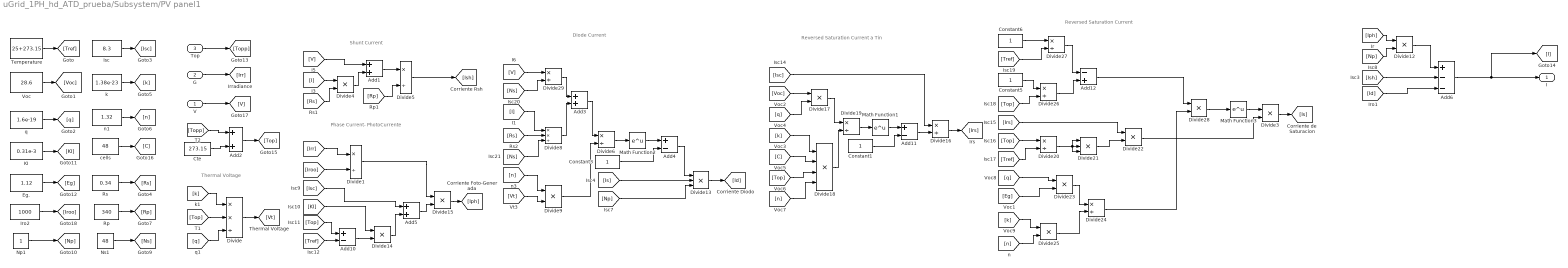
== system uGrid_1PH_hd_ATD_prueba/Subsystem/PV panel1 ==
  note: Thermal Voltage
  note: Shunt Current
  note: Phase Current- PhotoCurrente
  note: Diode Current
  note: Reversed Saturation Current a Tin
  note: Reversed Saturation Current
  V : Inport
  G : Inport  Port=2
  Top : Inport  Port=3
  Add{1..3,5} (4 alike) : Sum
  Add10 : Sum  Inputs=+-
  Add11 : Sum  Inputs=+-
  Add12 : Sum  Inputs=-+
  Add4 : Sum  Inputs=+-
  Add6 : Sum  Inputs=+--
  Constant{1,3,5..6} (4 alike) : Constant
  Cte : Constant  Value=273.15
  Divide : Product  Inputs=**/
  Divide{1,5..6,16,19..20,24,26..27,29} (10 alike) : Product  Inputs=*/
  Divide{3..4,9,12,14..15,17,22..23,25,28} (11 alike) : Product  Inputs=**
  Divide13 : Product  Inputs=***
  Divide18 : Product  Inputs=****
  Divide21 : Product  Inputs=***
  Divide8 : Product  Inputs=**/
  Eg. : Constant  Value=1.12
  Iro2 : Constant  Value=1000
  Isc : Constant  Value=8.3
  KI : Constant  Value=0.31e-3
  Math Function1 : Math  SaturateOnIntegerOverflow=on
  Math Function2 : Math  SaturateOnIntegerOverflow=on
  Math Function3 : Math  SaturateOnIntegerOverflow=on
  Np1 : Constant
  Ns1 : Constant  Value=48
  Rp : Constant  Value=340
  Rs : Constant  Value=0.34
  Temperature : Constant  Value=25+273.15
  Voc : Constant  Value=28.6
  cells : Constant  Value=48
  k : Constant  Value=1.38e-23
  n1 : Constant  Value=1.32
  q : Constant  Value=1.6e-19
  I : Outport
  wires:
  Temperature/1 -> [Tref]
  Voc/1 -> [Voc]
  q/1 -> [q]
  Isc/1 -> [Isc]
  k/1 -> [k]
  n1/1 -> [n]
  [k] -> Divide/1
  [Top] -> Divide/2
  [q] -> Divide/3
  Divide/1 -> [Vt]
  Divide3/1 -> [Is]
  [Ish] -> Add6/2
  Add6/1 -> I/1, [I]
  [I] -> Divide8/1
  [Rs] -> Divide8/2
  Divide8/1 -> Add3/2
  [n] -> Divide9/1
  [Vt] -> Divide9/2
  Divide9/1 -> Divide6/2
  Add3/1 -> Divide6/1
  Divide6/1 -> Math Function2/1
  Math Function2/1 -> Add4/1
  Add4/1 -> Divide13/1
  [Is] -> Divide13/2
  Divide13/1 -> [Id]
  Divide4/1 -> Add1/2
  Add1/1 -> Divide5/1
  [Rp] -> Divide5/2
  Divide5/1 -> [Ish]
  [Rs] -> Divide4/2
  [I] -> Divide4/1
  KI/1 -> [KI]
  Eg./1 -> [Eg]
  [V] -> Add1/1
  [Np] -> Divide13/3
  [Iph] -> Divide12/1
  [Np] -> Divide12/2
  Divide12/1 -> Add6/1
  [Isc] -> Add5/1
  [Top] -> Add10/1
  [Tref] -> Add10/2
  Add10/1 -> Divide14/2
  [KI] -> Divide14/1
  [Voc] -> Divide17/1
  [q] -> Divide17/2
  [k] -> Divide18/1
  [C] -> Divide18/2
  [Top] -> Divide18/3
  [n] -> Divide18/4
  Divide17/1 -> Divide19/1
  Divide18/1 -> Divide19/2
  Divide19/1 -> Math Function1/1
  Constant1/1 -> Add11/2
  Math Function1/1 -> Add11/1
  Add11/1 -> Divide16/2
  Divide16/1 -> [Irs]
  [Tref] -> Divide20/2
  [Top] -> Divide20/1
  Divide20/1 -> Divide21/2, Divide21/1, Divide21/3
  Divide21/1 -> Divide22/2
  [Irs] -> Divide22/1
  [q] -> Divide23/1
  Divide23/1 -> Divide24/1
  [k] -> Divide25/1
  [n] -> Divide25/2
  Divide25/1 -> Divide24/2
  Constant5/1 -> Divide26/1
  [Top] -> Divide26/2
  Constant6/1 -> Divide27/1
  [Tref] -> Divide27/2
  Divide27/1 -> Add12/1
  Divide26/1 -> Add12/2
  Add12/1 -> Divide28/1
  Divide24/1 -> Divide28/2
  Divide28/1 -> Math Function3/1
  Divide29/1 -> Add3/1
  [Ns] -> Divide29/2
  [V] -> Divide29/1
  [Ns] -> Divide8/3
  Divide14/1 -> Add5/2
  Add5/1 -> Divide15/2
  Divide15/1 -> [Iph]
  V/1 -> [V]
  G/1 -> [Irr]
  Top/1 -> [Topp]
  cells/1 -> [C]
  [Id] -> Add6/3
  Cte/1 -> Add2/2
  Add2/1 -> [Top]
  [Topp] -> Add2/1
  [Irr] -> Divide1/1
  [Iroo] -> Divide1/2
  Divide1/1 -> Divide15/1
  Iro2/1 -> [Iroo]
  Rs/1 -> [Rs]
  Rp/1 -> [Rp]
  Ns1/1 -> [Ns]
  Np1/1 -> [Np]
  Constant3/1 -> Add4/2
  [Isc] -> Divide16/1
  Math Function3/1 -> Divide3/1
  Divide22/1 -> Divide3/2
  [Eg] -> Divide23/2

== system uGrid_1PH_hd_ATD_prueba/1Ph_Inverter_bio/Subsystem/Steper1 ==
  In1 : Inport
  Product : Product
  Step : Step  Time=st_time  SampleTime=samp_f
  Out1 : Outport
  wires:
  Step/1 -> Product/2
  In1/1 -> Product/1
  Product/1 -> Out1/1

== system uGrid_1PH_hd_ATD_prueba/1Ph_Inverter_bio/Subsystem/Steper3 ==
  In1 : Inport
  Product : Product
  Step : Step  Time=st_time  SampleTime=samp_f
  Out1 : Outport
  wires:
  Product/1 -> Out1/1
  In1/1 -> Product/1
  Step/1 -> Product/2

== system uGrid_1PH_hd_ATD_prueba/1Ph_Inverter_diesel/Subsystem/Steper1 ==
  In1 : Inport
  Product : Product
  Step : Step  Time=st_time  SampleTime=samp_f
  Out1 : Outport
  wires:
  Product/1 -> Out1/1
  In1/1 -> Product/1
  Step/1 -> Product/2

== system uGrid_1PH_hd_ATD_prueba/1Ph_Inverter_diesel/Subsystem/Steper3 ==
  In1 : Inport
  Product : Product
  Step : Step  Time=st_time  SampleTime=samp_f
  Out1 : Outport
  wires:
  Step/1 -> Product/2
  In1/1 -> Product/1
  Product/1 -> Out1/1

== matlab function uGrid_1PH_hd_ATD_prueba/1Ph_Inverter_diesel/Subsystem/not_pwm ==
  data: u input; y output
function y = fcn(u)
%#codegen

if(u==0 || u<0)
    a=15;
else
    a=0;
end;

y = a;

== matlab function uGrid_1PH_hd_ATD_prueba/1Ph_Inverter_bio/Subsystem/not_pwm ==
  data: u input; y output
function y = fcn(u)
%#codegen

if(u==0 || u<0)
    a=15;
else
    a=0;
end;

y = a;

== matlab function uGrid_1PH_hd_ATD_prueba/LinearProg ==
  data: P_load input; Pbo output; P_e_alt input; kb input; kd input; PdMax input; PbMax input; Pdo output; P_e_alt_min input
function [Pbo, Pdo] = fcn(P_load, P_e_alt, kb, kd, PdMax, PbMax, P_e_alt_min)

% P_load es la potencia que se requiere en la carga.

% P_e_alt es la potencia estimada de generacion de las energias
% alternativas

% kb y kd son los pesos de las funcion de costo.

% las salidas son las potencias optimas para bio y diesel

Pb=0;
Pd=0;

D_P_e_alt = P_e_alt - P_e_alt_min; % superaavit de energia alternativa.

flagDelt = 0;

if(D_P_e_alt >= P_load)
    flagDelt = 1;
end
   

if(flagDelt==0)
    P_trad = P_load - D_P_e_alt;
    % flag: variable que indica si tiene sentido evaluar los
    % if's que se encuentran mas adelante. es decir, si flag = 0 
    % despues del primer if entonces NO se le esta pidiendo al sistema
    % mas potencia de la que puede generar y portanto el problema de 
    % optimizacion lineal tiene sentido.
    % entonces 
    flag=0;

    if(P_trad>PdMax+PbMax)
        Pd=PdMax;
        Pb=PbMax;
        flag=1;
    end

    % si ambas energias tienen el mismo factor de costo.
    if(kd==kb && flag==0)
        Pb=P_trad/2;
        Pd=P_trad/2;
    end

    % si la energia diesel es mas cara que la biomasa.
    if(kd>kb && flag==0)
        if(P_trad<=PbMax)
            Pb=P_trad;
            Pd=0;
        else
            Pb=PbMax;
            Pd=P_trad-PbMax;
        end
    end

    % si la biomasa es mas cara que la diesel.
    if(kd<kb && flag==0)
        if(P_trad<=PdMax)
            Pd=P_trad;
            Pb=0;
        else
            Pd=PdMax;
            Pb=P_trad-PdMax;
        end
    end
end

Pbo=Pb;
Pdo=Pd;

== matlab function uGrid_1PH_hd_ATD_prueba/MPC Controller/MPC_MatCalc1 ==
  data: ref input; PQ input; Hv output; F output; A output; lb output; ub output; lbA output; ubA output; Du input; MPCout input; G input; GF input
function [Hv, F, A, lb, ub, lbA, ubA] = MPC(ref, PQ, Du, MPCout, G, GF)

%%parametros del MPC


p = 100; % horizonte de prediccion
Nu = 100; % horizonte de control


%% Calculo de la salida de control.

H = G'*G+eye(2*Nu)*3000; % parte cuadratica del qp

ym = [ ones(p, 1)*PQ(1); ones(p, 1)*PQ(2) ]; % vector de la medida de tempearatura actual.

w = [ ones(p, 1)*ref(1); ones(p, 1)*ref(2) ]; % vector señal setpoint.

L = GF*Du+ym; % respuesta libre.

F = 2*(L-w)'*G; % parte lineal del problema qp.

A = zeros(1, 4*Nu*Nu);

lbA = zeros(1, 2*Nu);

ubA = zeros(1, 2*Nu);

Hv = M2V(H);

hip = HiBound(MPCout(1), 600, 10);
hiq = HiBound(MPCout(2), 5000, 1000);

lop = LowBound(MPCout(1), -100, -10);
loq = LowBound(MPCout(2), -100, -1000);

lb = [ones(1, Nu)*lop ones(1, Nu)*loq];
ub = [ones(1, Nu)*hip ones(1, Nu)*hiq];
end

% el control mpc implementado halla mediante programacion cuadratica
% los delta de u optimos deacuerdo a la funcion de coste. por este motivo
% es necesario implementar una logica adicional que permita limitar
% los valores de u (la salida) ya que estos no se manupilan directamente
% en el problema de programacion cuadratica.

% esta logica se implementan en las dos funciones locales que se encuentran
% a continuacion. una funcion define el limite superior y otra funcion para
% definir el limite inferior de los deltas de u deacuerdo al valor actual
% de u para asegurar que tanto los deltas de u como el valor de u esten
% limitados.
% esta funcion solo es correcta si max y Dmax son valores positivos.
function y = HiBound(X, max, Dmax)
    if(X>=0) % si la potencia X es positiva:
        if(max >= X)% si X no ha superado la potencia maxima:
            if(max-X >= Dmax) % si la distancia supera el cambio maximo deseado
                r = Dmax;
            else % si es menor al cambio maximo deseado
                r = max-X;
            end
        else % si X supera la potencia maxima deseada
            r = 0; % el delta maximo es 0 para que no se incremente mas.
        end
    else % si la potencia X es negativa, el incremento maximo es
        r = Dmax;
    end
    y = r;
end

% esta funcion para el lower bound se penso para trbajar con valores
% negativos. si min y Dmin no es negativo la funcion no funciona
% correctamente.
function y = LowBound(X, minv, Dmin)
    if(X<=0) % si la potencia X esta en el cuadrante inferior:
        if(minv <= X)% si X es mayor que la potencia minima:
            if(minv-X <= Dmin) % si la distancia supera el cambio maximo deseado
                r = Dmin;
            else % si es mayor al cambio maximo deseado
                r = minv-X;
            end
        else % si X es menor la potencia maxima deseada
            r = 0; % el delta maximo es 0 para que no se decremente mas.
        end
    else % si la potencia X es positiva, el decremento maximo es
        r = Dmin;
    end
    y = r;
end

== matlab function uGrid_1PH_hd_ATD_prueba/MPC Controller/MPC_OutLogic1 ==
  data: MPCout output; duv input; Duv output
function [MPCout, Duv] = MPC_out_Logic(duv)

%%parametros del MPC
Nu = 100; % horizonte de control.


%% variables del MPC
persistent Du; % deltas de u 
persistent out; % salida actual del conrolador MPC.

if isempty(Du) % inicializacion de los deltas de uu
    Du = zeros(2*Nu, 1);
end

if isempty(out) % inicializaion de la salida del controlador MPC
    out = [0; 0];
end


du = [duv(1), duv(Nu+1)];


Du = [du(1); Du(1:Nu-1); du(2); Du(Nu+1:end-1)];% actualizar historial deltas de u.

out = [ out(1)+du(1); out(2)+du(2) ]; %calcular salida del controlador.

MPCout = out;
Duv = Du;

== matlab function uGrid_1PH_hd_ATD_prueba/MPC Controller/MPC_MatCalc ==
  data: ref input; PQ input; Hv output; F output; A output; lb output; ub output; lbA output; ubA output; Du input; MPCout input; G input; GF input
function [Hv, F, A, lb, ub, lbA, ubA] = MPC(ref, PQ, Du, MPCout, G, GF)

%%parametros del MPC


p = 100; % horizonte de prediccion
Nu = 100; % horizonte de control


%% Calculo de la salida de control.

H = G'*G+eye(2*Nu)*3000; % parte cuadratica del qp

ym = [ ones(p, 1)*PQ(1); ones(p, 1)*PQ(2) ]; % vector de la medida de tempearatura actual.

w = [ ones(p, 1)*ref(1); ones(p, 1)*ref(2) ]; % vector señal setpoint.

L = GF*Du+ym; % respuesta libre.

F = 2*(L-w)'*G; % parte lineal del problema qp.

A = zeros(1, 4*Nu*Nu);

lbA = zeros(1, 2*Nu);

ubA = zeros(1, 2*Nu);

Hv = M2V(H);

hip = HiBound(MPCout(1), 600, 10);
hiq = HiBound(MPCout(2), 5000, 1000);

lop = LowBound(MPCout(1), -100, -10);
loq = LowBound(MPCout(2), -100, -1000);

lb = [ones(1, Nu)*lop ones(1, Nu)*loq];
ub = [ones(1, Nu)*hip ones(1, Nu)*hiq];
end

% el control mpc implementado halla mediante programacion cuadratica
% los delta de u optimos deacuerdo a la funcion de coste. por este motivo
% es necesario implementar una logica adicional que permita limitar
% los valores de u (la salida) ya que estos no se manupilan directamente
% en el problema de programacion cuadratica.

% esta logica se implementan en las dos funciones locales que se encuentran
% a continuacion. una funcion define el limite superior y otra funcion para
% definir el limite inferior de los deltas de u deacuerdo al valor actual
% de u para asegurar que tanto los deltas de u como el valor de u esten
% limitados.
% esta funcion solo es correcta si max y Dmax son valores positivos.
function y = HiBound(X, max, Dmax)
    if(X>=0) % si la potencia X es positiva:
        if(max >= X)% si X no ha superado la potencia maxima:
            if(max-X >= Dmax) % si la distancia supera el cambio maximo deseado
                r = Dmax;
            else % si es menor al cambio maximo deseado
                r = max-X;
            end
        else % si X supera la potencia maxima deseada
            r = 0; % el delta maximo es 0 para que no se incremente mas.
        end
    else % si la potencia X es negativa, el incremento maximo es
        r = Dmax;
    end
    y = r;
end

% esta funcion para el lower bound se penso para trbajar con valores
% negativos. si min y Dmin no es negativo la funcion no funciona
% correctamente.
function y = LowBound(X, minv, Dmin)
    if(X<=0) % si la potencia X esta en el cuadrante inferior:
        if(minv <= X)% si X es mayor que la potencia minima:
            if(minv-X <= Dmin) % si la distancia supera el cambio maximo deseado
                r = Dmin;
            else % si es mayor al cambio maximo deseado
                r = minv-X;
            end
        else % si X es menor la potencia maxima deseada
            r = 0; % el delta maximo es 0 para que no se decremente mas.
        end
    else % si la potencia X es positiva, el decremento maximo es
        r = Dmin;
    end
    y = r;
end

== matlab function uGrid_1PH_hd_ATD_prueba/MPC Controller/MPC_OutLogic ==
  data: MPCout output; duv input; Duv output
function [MPCout, Duv] = MPC_out_Logic(duv)

%%parametros del MPC
Nu = 100; % horizonte de control.


%% variables del MPC
persistent Du; % deltas de u 
persistent out; % salida actual del conrolador MPC.

if isempty(Du) % inicializacion de los deltas de uu
    Du = zeros(2*Nu, 1);
end

if isempty(out) % inicializaion de la salida del controlador MPC
    out = [0; 0];
end


du = [duv(1), duv(Nu+1)];


Du = [du(1); Du(1:Nu-1); du(2); Du(Nu+1:end-1)];% actualizar historial deltas de u.

out = [ out(1)+du(1); out(2)+du(2) ]; %calcular salida del controlador.

MPCout = out;
Duv = Du;

== matlab function uGrid_1PH_hd_ATD_prueba/1Ph_Inverter_bio1/not_pwm ==
  data: u input; y output
function y = fcn(u)
%#codegen

if(u==0 || u<0)
    a=15;
else
    a=0;
end;

y = a;

== matlab function uGrid_1PH_hd_ATD_prueba/LinearProg1 ==
  data: Q_load input; Qbo output; Q_e_alt input; kb input; kd input; QdMax input; QbMax input; Qdo output; Q_e_alt_min input
function [Qbo, Qdo] = fcn(Q_load, Q_e_alt, kb, kd, QdMax, QbMax, Q_e_alt_min)

% Q_load es la Qotencia que se requiere en la carga.

% Q_e_alt es la Qotencia estimada de generacion de las energias
% alternativas

% kb y kd son los Qesos de las funcion de costo.

% las salidas son las Qotencias oQtimas Qara bio y diesel

Qb=0;
Qd=0;

D_Q_e_alt = Q_e_alt - Q_e_alt_min; % suQeraavit de energia alternativa.

flagDelt = 0;

if(D_Q_e_alt >= Q_load)
    flagDelt = 1;
end
   

if(flagDelt==0)
    Q_trad = Q_load - D_Q_e_alt;
    % flag: variable que indica si tiene sentido evaluar los
    % if's que se encuentran mas adelante. es decir, si flag = 0 
    % desQues del Qrimer if entonces NO se le esta Qidiendo al sistema
    % mas Qotencia de la que Quede generar y Qortanto el Qroblema de 
    % oQtimizacion lineal tiene sentido.
    % entonces 
    flag=0;

    if(Q_trad>QdMax+QbMax)
        Qd=QdMax;
        Qb=QbMax;
        flag=1;
    end

    % si ambas energias tienen el mismo factor de costo.
    if(kd==kb && flag==0)
        Qb=Q_trad/2;
        Qd=Q_trad/2;
    end

    % si la energia diesel es mas cara que la biomasa.
    if(kd>kb && flag==0)
        if(Q_trad<=QbMax)
            Qb=Q_trad;
            Qd=0;
        else
            Qb=QbMax;
            Qd=Q_trad-QbMax;
        end
    end

    % si la biomasa es mas cara que la diesel.
    if(kd<kb && flag==0)
        if(Q_trad<=QdMax)
            Qd=Q_trad;
            Qb=0;
        else
            Qd=QdMax;
            Qb=Q_trad-QdMax;
        end
    end
end

Qbo=Qb;
Qdo=Qd;
